simulink model "extGaWithSwitch"  (R2012b)
settings: Solver=ode3  StartTime=0.0  StopTime=inf  FixedStep=0.001  RelTol=1e-3
undefined symbols (not defined in the file): HIL, qc_get_step_size
libraries: quarc_library x5
settings Model: SimulationMode=external  ExtModeTrigDuration=50000  Creator=anzhuan  LastModifiedBy=anzhuan
settings SolverCC: PositivePriorityOrder=on
settings RTWCC: SystemTargetFile=quarc_win64.tlc  TemplateMakefile=quarc_default_tmf  Description=QUARC Win64 Target  ProcessScript=quarc_win64_make_rtw_hook
settings STFCustomTargetCC: TargetPreCompLibLocation=C:\PROGRA~3\QUARC\lib\2012b\win64\release  CodeReplacementLibrary=ANSI_C  GeneratePreprocessorConditionals=Disable all  CombineOutputUpdateFcns=on  GRTInterface=off  SystemTargetFile=quarc_win64.tlc
settings GRTTargetCC: TargetPreCompLibLocation=C:\PROGRA~3\QUARC\lib\2012b\win64\release  ParMdlRefBuildCompliant=off  CompOptLevelCompliant=off  ConcurrentExecutionCompliant=off  MatFileLogging=off  ExtMode=on  ExtModeMexFile=quarc_comm

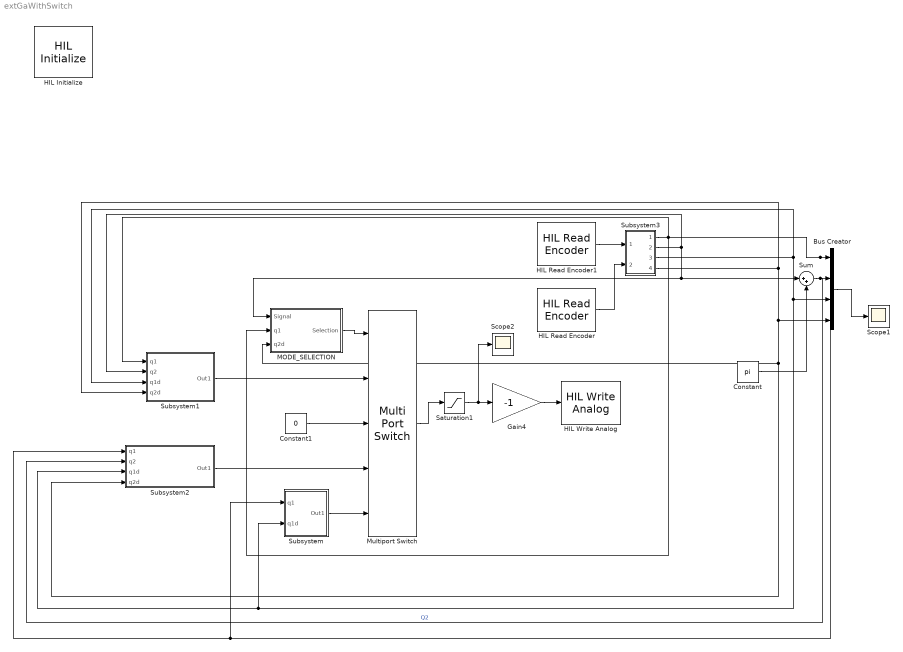
== system extGaWithSwitch ==
  Bus Creator : BusCreator
  Constant : Constant  Value=pi
  Constant1 : Constant  Value=0
  Gain4 : Gain  Gain=-1
  HIL Initialize : quarc_library/Data Acquisition/Generic/Configuration/HIL Initialize  Priority=-99  object_name=HIL-1  board_type=q2_usb  board_number=0  board_options=d0=digital;d1=digital;led=auto;update_rate=normal;decimation=1  exclusive=off  active=off  hardware_clocks=[0]  clock_modes=[]  initial_clock_frequencies=[]  set_clock_params_at_start=off  set_clock_params_at_switch_in=off  set_clock_frequencies_at_start=off  set_clock_frequencies_at_switch_in=off  analog_input_channels=[0:1]  analog_input_maximums=10  analog_input_minimums=-10  set_analog_input_params_at_start=on  set_analog_input_params_at_switch_in=off  analog_output_channels=[0:1]  analog_output_maximums=10  analog_output_minimums=-10  initial_analog_outputs=[0]  final_analog_outputs=[0]  watchdog_analog_outputs=0  set_analog_output_params_at_start=on  set_analog_output_params_at_switch_in=off  set_analog_outputs_at_start=on  set_analog_outputs_at_switch_in=off  set_analog_outputs_at_terminate=on  set_analog_outputs_at_switch_out=off  set_analog_outputs_on_watchdog=off  digital_input_channels=[]  digital_output_channels=[]  digital_output_configuration=[]  initial_digital_outputs=[1]  final_digital_outputs=[1]  watchdog_digital_outputs=[1]  set_digital_output_params_at_start=off  set_digital_output_params_at_switch_in=off  set_digital_outputs_at_start=on  set_digital_outputs_at_switch_in=off  set_digital_outputs_at_terminate=on  set_digital_outputs_at_switch_out=off  set_digital_outputs_on_watchdog=off  encoder_channels=[0:1]  quadrature=[4]  encoder_filter_frequency=[]  initial_encoder_counts=[0]  set_encoder_params_at_start=on  set_encoder_params_at_switch_in=off  set_encoder_counts_at_start=on  set_encoder_counts_at_switch_in=off  pwm_channels=[]  pwm_modes=[0]  pwm_frequency=1/0.020  pwm_configuration=[]  pwm_alignment=[]  pwm_polarity=[]  pwm_leading_deadband=[]  pwm_trailing_deadband=[]  initial_pwm_outputs=[0]  final_pwm_outputs=[0]  watchdog_pwm_outputs=[0]  set_pwm_params_at_start=on  set_pwm_params_at_switch_in=off  set_pwm_outputs_at_start=on  set_pwm_outputs_at_switch_in=off  set_pwm_outputs_at_terminate=on  set_pwm_outputs_at_switch_out=off  set_pwm_outputs_on_watchdog=off  other_output_channels=[]  initial_other_outputs=[]  final_other_outputs=[]  watchdog_other_outputs=[]  set_other_outputs_at_start=off  set_other_outputs_at_switch_in=off  set_other_outputs_at_terminate=off  set_other_outputs_at_switch_out=off  set_other_outputs_on_watchdog=off
  HIL Read Encoder : quarc_library/Data Acquisition/Generic/Immediate I//O/HIL Read Encoder  object_name=HIL-1  channels=1  sample_time=qc_get_step_size  active=on  vector_output=off  data_type_mode=Inherit via back propagation  data_type=double
  HIL Read Encoder1 : quarc_library/Data Acquisition/Generic/Immediate I//O/HIL Read Encoder  object_name=HIL-1  channels=0  sample_time=qc_get_step_size  active=on  vector_output=off  data_type_mode=Inherit via back propagation  data_type=double
  HIL Write Analog : quarc_library/Data Acquisition/Generic/Immediate I//O/HIL Write Analog  object_name=HIL-1  channels=0  sample_time=-1  active=off  vector_input=off
  MODE_SELECTION : Subsystem
  Multiport Switch : MultiPortSwitch  Inputs=4
  Saturation1 : Saturate  UpperLimit=10  LowerLimit=-10
  Scope1 : Scope
      settings: ShowLegends=on  YMin=-1.5  YMax=10  SaveName=states
  Scope2 : Scope
      settings: ShowLegends=on  YMin=-22.5  YMax=20  SaveName=V1
  Subsystem : Subsystem
  Subsystem1 : Subsystem
  Subsystem2 : Subsystem
  Subsystem3 : Subsystem
  Sum : Sum  Inputs=|++
  wires:
  Bus Creator/1 -> Scope1/1
  Constant/1 -> Sum/2
  Sum/1 -> Bus Creator/2, Subsystem2/2(q2)  "Q2"
  Multiport Switch/1 -> Saturation1/1
  Gain4/1 -> HIL Write Analog/1
  Saturation1/1 -> Scope2/1, Gain4/1
  Constant1/1 -> Multiport Switch/3
  MODE_SELECTION/1(Selection) -> Multiport Switch/1
  Subsystem1/1(Out1) -> Multiport Switch/2
  Subsystem2/1(Out1) -> Multiport Switch/4
  Subsystem/1(Out1) -> Multiport Switch/5
  Subsystem3/2(Out2) -> Sum/1, MODE_SELECTION/1(Signal), Subsystem1/2(q2)
  Subsystem3/4(Out4) -> Subsystem2/4(q2d), MODE_SELECTION/3(q2d), Bus Creator/4, Subsystem1/4(q2d)
  Subsystem3/1(Out1) -> Subsystem1/1(q1), Subsystem/1(q1), Subsystem2/1(q1), Bus Creator/1, MODE_SELECTION/2(q1)
  Subsystem3/3(Out3) -> Bus Creator/3, Subsystem/2(q1d), Subsystem2/3(q1d), Subsystem1/3(q1d)
  HIL Read Encoder1/1 -> Subsystem3/1(In1)
  HIL Read Encoder/1 -> Subsystem3/2(In2)

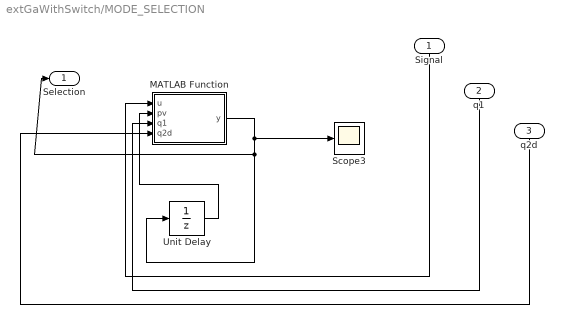
== system extGaWithSwitch/MODE_SELECTION ==
  Signal : Inport
  q1 : Inport  Port=2
  q2d : Inport  Port=3
  MATLAB Function : MATLAB Function  TreatAsAtomicUnit=on
  Scope3 : Scope
      settings: ShowLegends=on  YMin=-22.5  YMax=20  SaveName=V
  Unit Delay : UnitDelay  SampleTime=-1
  Selection : Outport
  wires:
  MATLAB Function/1(y) -> Selection/1, Unit Delay/1, Scope3/1
  Unit Delay/1 -> MATLAB Function/2(pv)
  Signal/1 -> MATLAB Function/1(u)
  q1/1 -> MATLAB Function/3(q1)
  q2d/1 -> MATLAB Function/4(q2d)

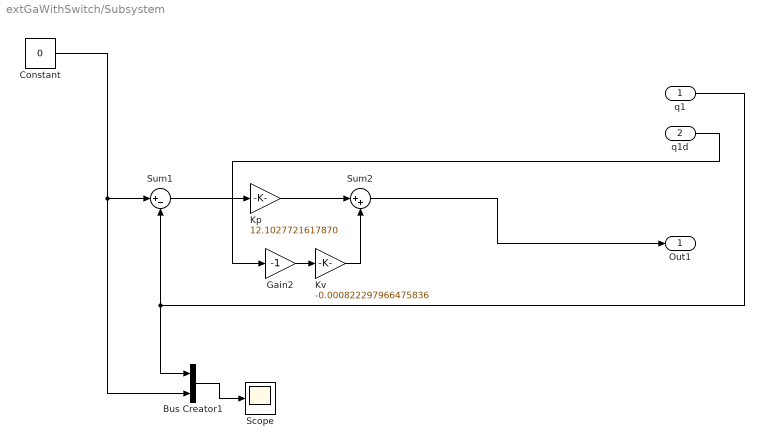
== system extGaWithSwitch/Subsystem ==
  q1 : Inport
  q1d : Inport  Port=2
  Bus Creator1 : BusCreator  Inputs=2
  Constant : Constant  Value=0
  Gain2 : Gain  Gain=-1
  Kp : Gain  Gain=12.1027721617870
  Kv : Gain  Gain=-0.000822297966475836
  Scope : Scope
      settings: ShowLegends=on  SaveName=ScopeData3
  Sum1 : Sum  Inputs=|+-
  Sum2 : Sum  Inputs=|++
  Out1 : Outport
  wires:
  q1d/1 -> Gain2/1
  Kp/1 -> Sum2/1
  Sum1/1 -> Kp/1
  Gain2/1 -> Kv/1
  Kv/1 -> Sum2/2
  Sum2/1 -> Out1/1
  Bus Creator1/1 -> Scope/1
  Constant/1 -> Sum1/1, Bus Creator1/2
  q1/1 -> Sum1/2, Bus Creator1/1

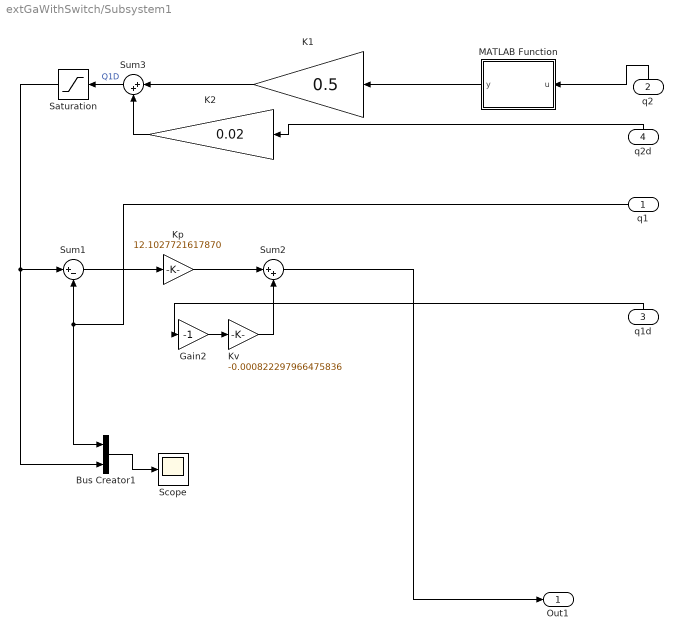
== system extGaWithSwitch/Subsystem1 ==
  q1 : Inport
  q2 : Inport  Port=2
  q1d : Inport  Port=3
  q2d : Inport  Port=4
  Bus Creator1 : BusCreator  Inputs=2
  Gain2 : Gain  Gain=-1
  K1 : Gain  Gain=0.5
  K2 : Gain  Gain=0.02
  Kp : Gain  Gain=12.1027721617870
  Kv : Gain  Gain=-0.000822297966475836
  MATLAB Function : MATLAB Function  TreatAsAtomicUnit=on
  Saturation : Saturate
  Scope : Scope
      settings: ShowLegends=on
  Sum1 : Sum  Inputs=|+-
  Sum2 : Sum  Inputs=|++
  Sum3 : Sum  Inputs=|++
  Out1 : Outport
  wires:
  q1d/1 -> Gain2/1
  q2d/1 -> K2/1
  Kp/1 -> Sum2/1
  Sum1/1 -> Kp/1
  Gain2/1 -> Kv/1
  Kv/1 -> Sum2/2
  Sum2/1 -> Out1/1
  K1/1 -> Sum3/1
  K2/1 -> Sum3/2
  Bus Creator1/1 -> Scope/1
  Sum3/1 -> Saturation/1  "Q1D"
  Saturation/1 -> Sum1/1, Bus Creator1/2
  q2/1 -> MATLAB Function/1(u)
  MATLAB Function/1(y) -> K1/1
  q1/1 -> Bus Creator1/1, Sum1/2

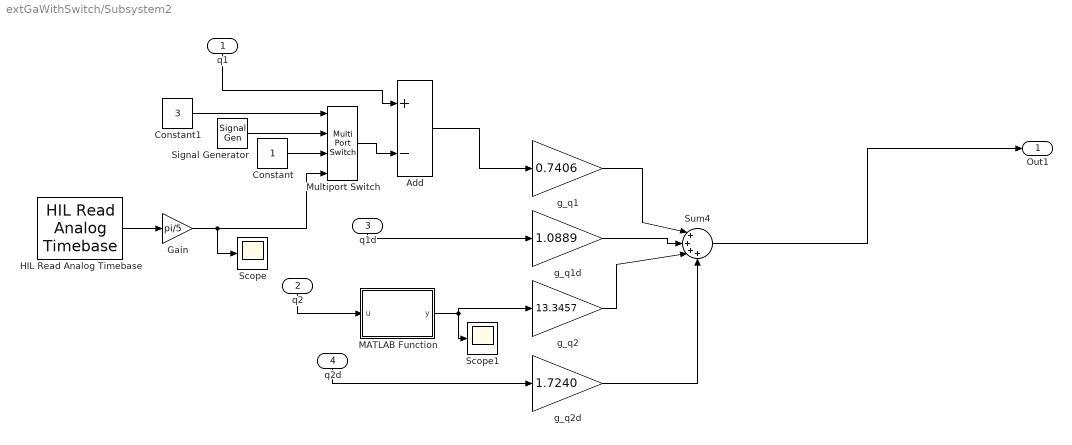
== system extGaWithSwitch/Subsystem2 ==
  q1 : Inport
  q2 : Inport  Port=2
  q1d : Inport  Port=3
  q2d : Inport  Port=4
  Add : Sum  Inputs=+-
  Constant : Constant
  Constant1 : Constant  Value=3
  Gain : Gain  Gain=pi/5
  HIL Read Analog Timebase : quarc_library/Data Acquisition/Generic/Timebases/HIL Read Analog Timebase  object_name=HIL-1  clock=0  channels=0  samples_in_buffer=max(ceil(1/qc_get_step_size), 1)  active=on  vector_output=off
      settings: AttributesFormatString=(%<object_name>)
  MATLAB Function : MATLAB Function  TreatAsAtomicUnit=on
  Multiport Switch : MultiPortSwitch
  Scope : Scope
  Scope1 : Scope
      settings: SaveName=ScopeData2
  Signal Generator : SignalGenerator  Frequency=0.1  Units=rad/sec
  Sum4 : Sum  Inputs=|++++
  g_q1 : Gain  Gain=0.7406
  g_q1d : Gain  Gain=1.0889
  g_q2 : Gain  Gain=13.3457
  g_q2d : Gain  Gain=1.7240
  Out1 : Outport
  wires:
  q1/1 -> Add/1
  q2d/1 -> g_q2d/1
  q1d/1 -> g_q1d/1
  g_q1/1 -> Sum4/1
  g_q1d/1 -> Sum4/2
  g_q2/1 -> Sum4/3
  g_q2d/1 -> Sum4/4
  Sum4/1 -> Out1/1
  Signal Generator/1 -> Multiport Switch/2
  Add/1 -> g_q1/1
  Constant/1 -> Multiport Switch/3
  Multiport Switch/1 -> Add/2
  HIL Read Analog Timebase/1 -> Gain/1
  Constant1/1 -> Multiport Switch/1
  Gain/1 -> Multiport Switch/4, Scope/1
  q2/1 -> MATLAB Function/1(u)
  MATLAB Function/1(y) -> g_q2/1, Scope1/1

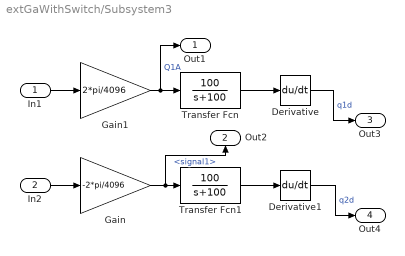
== system extGaWithSwitch/Subsystem3 ==
  In1 : Inport
  In2 : Inport  Port=2
  Derivative : Derivative
  Derivative1 : Derivative
  Gain : Gain  Gain=-2*pi/4096
  Gain1 : Gain  Gain=2*pi/4096
  Transfer Fcn : TransferFcn  Numerator=[100]  Denominator=[1 100]
  Transfer Fcn1 : TransferFcn  Numerator=[100]  Denominator=[1 100]
  Out1 : Outport
  Out2 : Outport  Port=2
  Out3 : Outport  Port=3
  Out4 : Outport  Port=4
  wires:
  In2/1 -> Gain/1
  In1/1 -> Gain1/1
  Gain1/1 -> Transfer Fcn/1, Out1/1  "Q1A"
  Transfer Fcn1/1 -> Derivative1/1
  Transfer Fcn/1 -> Derivative/1
  Derivative/1 -> Out3/1  "q1d"
  Derivative1/1 -> Out4/1  "q2d"
  Gain/1 -> Out2/1, Transfer Fcn1/1  "<signal1>"

== matlab function extGaWithSwitch/Subsystem2/MATLAB Function ==
  data: u input; y output
function y = fcn(u)
%#codegen
x=sin(u);
x2=cos(u);
y=atan2(x,x2);
end

== matlab function extGaWithSwitch/MODE_SELECTION/MATLAB Function ==
  data: u input; y output; pv input; q1 input; q2d input
function y = angle(u,pv,q1,q2d)
%#codegen

y=1;


u1 = atan2(sin(u),cos(u))

%u
if u1<= 10 /180*pi && u1>= -10 /180*pi
    if pv == 0
        y = 1;
    elseif pv == 4 && q2d>=-0.1 && q2d <= 0.1 && q1 == 0
        y = 1;
    elseif pv == 2 && q2d>=-0.3 && q2d <= 0.3
        y = 4;
    else 
        y = pv;
    end
elseif u1>10/180*pi && u1<=155/180*pi || u1<-10/180*pi && u1 >=-155/180*pi 
    if pv == 3
        y = 2;
    else
        y = pv;
    end
elseif u1>155/180*pi && u1<=pi || u1<-155/180*pi && u1>=-1*pi
    if pv == 1
        y = 3;
    else
        y = pv;
    end
end

end

== matlab function extGaWithSwitch/Subsystem1/MATLAB Function ==
  data: u input; y output
function y = fcn(u)
%#codegen
x=sin(u);
x2=cos(u);
y=atan2(x,x2);
end
